simulink model "Commande_en_position"  (R2018a)
settings: Solver=VariableStepAuto  StartTime=0.0  StopTime=10.0  RelTol=1e-3
values from neighbouring files (symbols this model uses):
  q_df = [ 0.00; 1.00;  0.00;  0.00;  0.00;  0.00]    [Q19Test.m]    (also in Q20Test.m)
  q_di = [-1.00; 0.00; -1.00; -1.00; -1.00; -1.00]    [Q19Test.m]    (also in Q20Test.m)
settings Model: Creator=Victor Kobayashi  LastModifiedBy=Victor Kobayashi

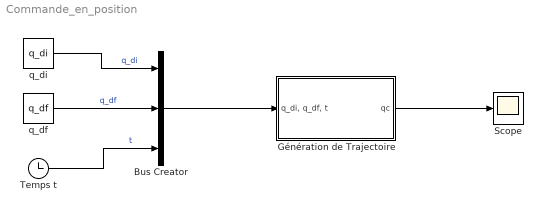
== system Commande_en_position ==
  Bus Creator : BusCreator  Inputs=3
  Génération de Trajectoire : Subsystem
  Scope : Scope
  "Temps t " : Clock
  "q_df " : Constant  Value=q_df
  q_di : Constant  Value=q_di
  wires:
  Génération de Trajectoire/1("qc ") -> Scope/1
  "q_df "/1 -> Bus Creator/2  "q_df"
  Bus Creator/1 -> Génération de Trajectoire/1("q_di, q_df, t ")
  q_di/1 -> Bus Creator/1  "q_di"
  "Temps t "/1 -> Bus Creator/3  "t"

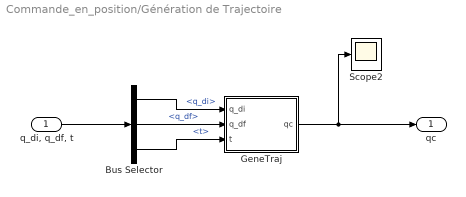
== system Commande_en_position/Génération de Trajectoire ==
  "q_di, q_df, t " : Inport
  Bus Selector : BusSelector  OutputSignals=q_di,q_df,t
  "GeneTraj " : MATLAB Function  TreatAsAtomicUnit=on
  Scope2 : Scope
  "qc " : Outport
  wires:
  "GeneTraj "/1(qc) -> Scope2/1, "qc "/1
  "q_di, q_df, t "/1 -> Bus Selector/1
  Bus Selector/1 -> "GeneTraj "/1(q_di)  "<q_di>"
  Bus Selector/2 -> "GeneTraj "/2(q_df)  "<q_df>"
  Bus Selector/3 -> "GeneTraj "/3(t)  "<t>"

== matlab function Commande_en_position/Génération de Trajectoire/GeneTraj  ==
  data: q_di input; qc output; q_df input; t input
function qc = fcn(q_di, q_df, t)

qc  = GeneTraj(q_di, q_df, t);
